simulink model "Scenario_2_v2"  (R2020b)
settings: Solver=ode1  StartTime=0.0  StopTime=10  FixedStep=Ts  MaxStep=Ts*2  MinStep=Ts/5  RelTol=1e-3
values from neighbouring files (symbols this model uses):
  c0 = c0_zeb    (= 6.57988e-09)    [Scenario_17_parameters_v2.m]    (also in Scenario_1_parameters_v2.m; Scenario_2_parameters_v2.m; Scenario_3_parameters_v2.m)
  c1 = c1_zeb    (= 9.15905e-09)    [Scenario_17_parameters_v2.m]    (also in Scenario_1_parameters_v2.m; Scenario_2_parameters_v2.m; Scenario_3_parameters_v2.m)
  fg = 50    [Scenario_17_parameters_v2.m]    (also in Scenario_1_parameters_v2.m; Scenario_2_parameters_v2.m; Scenario_3_parameters_v2.m)
  G1gen = 0.4692    [Scenario_17_parameters_v2.m]    (also in Scenario_1_parameters_v2.m = 0.1; Scenario_2_parameters_v2.m = 0.298581; Scenario_3_parameters_v2.m = 0.65)
  G2gen = 0.80    (= 0.8)    [Scenario_1_parameters_v2.m]    (also in Scenario_2_parameters_v2.m = 0.7; Scenario_3_parameters_v2.m = 0.4)
  G3gen = 0.85    [Scenario_1_parameters_v2.m]    (also in Scenario_2_parameters_v2.m = 0.9; Scenario_3_parameters_v2.m = 0.6)
  G4sgen = 0.8186    [Scenario_2_parameters_v2.m]
  G5gen = 0.75    [Scenario_17_parameters_v2.m]    (also in Scenario_1_parameters_v2.m = 0.8; Scenario_2_parameters_v2.m = 0.8; Scenario_3_parameters_v2.m = 0.705)
  G6gen = 0.90    (= 0.9)    [Scenario_17_parameters_v2.m]    (also in Scenario_1_parameters_v2.m; Scenario_2_parameters_v2.m = 0.81797; Scenario_3_parameters_v2.m = 0.45)
  G6sgen = 0.7    [Scenario_2_parameters_v2.m]
  G7gen = 0.20    (= 0.2)    [Scenario_17_parameters_v2.m]    (also in Scenario_1_parameters_v2.m = 0.5227; Scenario_2_parameters_v2.m = 0.5098; Scenario_3_parameters_v2.m = 0.4)
  Iovc = 1.2    [Scenario_17_parameters_v2.m]    (also in Scenario_1_parameters_v2.m; Scenario_2_parameters_v2.m; Scenario_3_parameters_v2.m)
  l0 = l0_zeb    (= 0.00368)    [Scenario_17_parameters_v2.m]    (also in Scenario_1_parameters_v2.m; Scenario_2_parameters_v2.m; Scenario_3_parameters_v2.m)
  l1 = l1_zeb    (= 0.00128)    [Scenario_17_parameters_v2.m]    (also in Scenario_1_parameters_v2.m; Scenario_2_parameters_v2.m; Scenario_3_parameters_v2.m)
  L3dem = 0.30    (= 0.3)    [Scenario_17_parameters_v2.m]    (also in Scenario_1_parameters_v2.m = 0.1; Scenario_2_parameters_v2.m = 0.1; Scenario_3_parameters_v2.m = 0.2)
  L4dem = 0.30    (= 0.3)    [Scenario_1_parameters_v2.m]    (also in Scenario_2_parameters_v2.m)
  L5dem = 0.25    [Scenario_17_parameters_v2.m]    (also in Scenario_1_parameters_v2.m = 0.35; Scenario_2_parameters_v2.m = 0.35; Scenario_3_parameters_v2.m = 0.1)
  L6dem = 0.15    [Scenario_1_parameters_v2.m]    (also in Scenario_2_parameters_v2.m; Scenario_3_parameters_v2.m = 0.1)
  L7dem = 0.10    (= 0.1)    [Scenario_1_parameters_v2.m]    (also in Scenario_2_parameters_v2.m; Scenario_3_parameters_v2.m = 0.2)
  Pr = Sr*PF    (= 1600500000)    [Scenario_17_parameters_v2.m]    (also in Scenario_1_parameters_v2.m = 1472500000; Scenario_2_parameters_v2.m = 1805000000; Scenario_3_parameters_v2.m = 12740000000)
  Qr = sqrt(Sr^2 - Pr^2)    [Scenario_17_parameters_v2.m]    (also in Scenario_1_parameters_v2.m; Scenario_2_parameters_v2.m; Scenario_3_parameters_v2.m)
  r0 = r0_zeb    (= 0.39362)    [Scenario_17_parameters_v2.m]    (also in Scenario_1_parameters_v2.m; Scenario_2_parameters_v2.m; Scenario_3_parameters_v2.m)
  r1 = r1_zeb    (= 0.06862)    [Scenario_17_parameters_v2.m]    (also in Scenario_1_parameters_v2.m; Scenario_2_parameters_v2.m; Scenario_3_parameters_v2.m)
  Rtpu = Xtpu/40    (= 0.0025)    [Scenario_17_parameters_v2.m]    (also in Scenario_1_parameters_v2.m = 0.00375; Scenario_2_parameters_v2.m = 0.00375; Scenario_3_parameters_v2.m)
  S1non = 700e6    (= 700000000)    [Scenario_17_parameters_v2.m]    (also in Scenario_1_parameters_v2.m = 400000000; Scenario_2_parameters_v2.m = 400000000; Scenario_3_parameters_v2.m = 1000000000)
  S2non = 300e6    (= 300000000)    [Scenario_1_parameters_v2.m]    (also in Scenario_2_parameters_v2.m; Scenario_3_parameters_v2.m = 3000000000)
  S3non = 200e6    (= 200000000)    [Scenario_1_parameters_v2.m]    (also in Scenario_2_parameters_v2.m; Scenario_3_parameters_v2.m = 1000000000)
  S4snon = 200e6    (= 200000000)    [Scenario_2_parameters_v2.m]
  S5non = 400e6    (= 400000000)    [Scenario_17_parameters_v2.m]    (also in Scenario_1_parameters_v2.m = 500000000; Scenario_2_parameters_v2.m = 500000000; Scenario_3_parameters_v2.m = 2000000000)
  S6non = 150e6    (= 150000000)    [Scenario_17_parameters_v2.m]    (also in Scenario_1_parameters_v2.m = 400000000; Scenario_2_parameters_v2.m = 400000000; Scenario_3_parameters_v2.m = 3000000000)
  S6snon = 200e6    (= 200000000)    [Scenario_2_parameters_v2.m]
  S7non = 1500e6    (= 1500000000)    [Scenario_17_parameters_v2.m]    (also in Scenario_1_parameters_v2.m = 200000000; Scenario_2_parameters_v2.m = 200000000; Scenario_3_parameters_v2.m = 4000000000)
  tonvsc = 0    [Scenario_17_parameters_v2.m]    (also in Scenario_1_parameters_v2.m; Scenario_2_parameters_v2.m; Scenario_3_parameters_v2.m = 0.0001)
  Ts = 50e-6    (= 5e-05)    [Scenario_17_parameters_v2.m]    (also in Scenario_1_parameters_v2.m = 0.0002; Scenario_2_parameters_v2.m = 2e-05; Scenario_3_parameters_v2.m = 0.0001)
  Vhv = 220e3    (= 220000)    [Scenario_17_parameters_v2.m]    (also in Scenario_1_parameters_v2.m; Scenario_2_parameters_v2.m; Scenario_3_parameters_v2.m)
  Vmv = 22e3    (= 22000)    [Scenario_17_parameters_v2.m]    (also in Scenario_1_parameters_v2.m; Scenario_2_parameters_v2.m; Scenario_3_parameters_v2.m)
  w_pll = 2*pi*80    (= 502.654824574)    [Scenario_17_parameters_v2.m]    (also in Scenario_1_parameters_v2.m; Scenario_2_parameters_v2.m; Scenario_3_parameters_v2.m)
  wc1 = wsw1/10    (= 848.230016469)    [Scenario_17_parameters_v2.m]    (also in Scenario_1_parameters_v2.m; Scenario_2_parameters_v2.m; Scenario_3_parameters_v2.m)
  wdc1 = wc1/10    (= 84.8230016469)    [Scenario_17_parameters_v2.m]    (also in Scenario_1_parameters_v2.m; Scenario_2_parameters_v2.m; Scenario_3_parameters_v2.m)
  wpq1 = wc1/10    (= 84.8230016469)    [Scenario_17_parameters_v2.m]    (also in Scenario_1_parameters_v2.m; Scenario_2_parameters_v2.m; Scenario_3_parameters_v2.m)
  wsw1 = ksw1*2*pi*fg    (= 8482.30016469)    [Scenario_17_parameters_v2.m]    (also in Scenario_1_parameters_v2.m; Scenario_2_parameters_v2.m; Scenario_3_parameters_v2.m)
  Xtpu = 0.10    (= 0.1)    [Scenario_17_parameters_v2.m]    (also in Scenario_1_parameters_v2.m = 0.15; Scenario_2_parameters_v2.m = 0.15; Scenario_3_parameters_v2.m)
undefined symbols (not defined in the file or in its folder): D11, Delta, Newton, Raphson
libraries: powerlib x214, simulink_extras x133, powerlib_meascontrol x102, pid_lib x48, simulink x32, eeTransforms x24, spsFirstOrderFilterLib x16, eePwmGeneratorTwoLevel x4
(part 2 of 19)

== system Scenario_2_v2/G2 ==
  Bus Selector : BusSelector  OutputSignals=Pabc,Qabc,vqp,vdp,vqn,vdn,iqp,idp,iqn,idn,f
  Constant : Constant  Value=S2non*G2gen
  Constant1 : Constant  Value=50e6
  Goto1 : Goto  Commented=on  GotoTag=Pg2  TagVisibility=global
  Goto3 : Goto  Commented=on  GotoTag=vdqpng2  TagVisibility=global
  Goto4 : Goto  Commented=on  GotoTag=idqpng2  TagVisibility=global
  Goto5 : Goto  Commented=on  GotoTag=Qg2  TagVisibility=global
  Mux2 : Mux
  Mux3 : Mux
  VSC v2 : Subsystem  mask{vscmod=EMT Average, fg=fg, Vhv=Vhv, Vmv=Vmv, Pconv=S2non, Rtpu=Rtpu, Xtpu=Xtpu, qmode=Active power, dmode=Reactive power, wsw=wsw1, wn_pll=w_pll, wc=wc1, wpq=wpq1, wdc=wdc1, koc=Iovc, Cdc=3100e-6, tfilt=1*(1/wsw1), negseq_en=on, fdroop_en=off, Vacdroop_en=off, LVRT_en=off, Kfdroop=0.05, fdroop_per=10, Kvdroop=0.1, Vacdroop_per=10, Vlvrt0=0.9, Vlvrt_min=0.5, Qmax_lvrt=0.9, V0pu=0.9540, theta0=-32.40, P0=S2non*G2gen, Q0=50e6}
      mask prompts: vscmod "VSC Model"; fg "AC grid frequency (Hz)"; Vhv "Grid-side voltage (V)(LL-rms)"; Vmv "Converter-side voltage (V)(LL-rms)"; Pconv "Converter nominal power (VA)"; Rtpu "Resistance seen by the converter (p.u)"; Xtpu "Reactance seen by the converter (p.u)"; qmode "q-axis control mode"; dmode "d-axis control mode"; wsw "Switching frequency (rad/s)"; wn_pll "PLL filter natural frequency"; wc "Current-control bandwidth (rad/s)"; wpq "PQ control bandwidth (rad/s)"; wdc "DC Voltage control bandwidth(rad/s)"; koc "Overcurrent factor (p.u)"; Cdc "DC-side total capacitance (F)"; tfilt "Vabc filter time constant (s)"; negseq_en "Enable negative sequence control"; fdroop_en "Enable frequency droop"; Vacdroop_en "Enable AC voltage droop"; LVRT_en "Enable LVRT"; Kfdroop "Frequency droop (p.u)"; fdroop_per "Percentage of converter power to contribute with droop (%)"; Kvdroop "Voltage droop (p.u)"; Vacdroop_per "Percentage of converter power to contribute with droop (%)"; Vlvrt0 "initial voltage (p.u)"; Vlvrt_min "minimum voltage (p.u)"; Qmax_lvrt "max power injected at min voltage (p.u)"; V0pu "Initial terminal voltage magnitude (pu)"; theta0 "Initial terminal voltage angle (deg)"; P0 "Initial active power (W)"; Q0 "Initial reactive power (VAr)"
      mask init:
      | %% ----------------------VSC Parameters-------------------------- %%
      | j = 1i;
      | r = Vhv/Vmv;                    % Transformer ratio
      | Vmvpk = Vmv*sqrt(2)/sqrt(3);    % Converter-side voltage phase-to-ground peak-to-peak
      | Vhvpk = Vhv*sqrt(2)/sqrt(3);    % Grid-side voltage phase-to-ground peak-to-peak  
      | Vdc = 2*Vhvpk;                  % Nominal DC voltage 
      | ksw = round(wsw/(2*pi*fg));      % Calculates switching ratio
      | Iconvbase = 2*Pconv/(3*Vmvpk);  % Converter base current (A)
      | Zbmv = Vmv^2/Pconv;             % Base voltage referred to the converter side
      | Imax = koc*Iconvbase;   % Converter maximum output current
      | %Cdc = 2*Hvsc*Pconv/Vdc^2;       % DC capacitor
      | 
      | Xt = Xtpu*Zbmv;        % p.u to (Ohms)
      | Lt = Xt/(2*pi*fg);              % p.u to (H)
      | Rt = Rtpu*Zbmv;        % p.u. to (Ohms)
      | 
      | % -------------LVRT--------------%
      | Klvrt = Qmax_lvrt/(Vlvrt_min-Vlvrt0); % Defines LVRT inclination of the V/I LVRT characteristic
      | 
      | % ------------ PLL ------------- %
      | zeta_pll = 1/sqrt(2);           % Damping
      | kp_pll = 2*zeta_pll*wn_pll/(Vmvpk);
      | tau_pll = 2*zeta_pll/wn_pll;
      | 
      | % ------------ Inner-loop (current control) ------------ %
      | kp_c = Lt*wc; 
      | ti_c = Lt/Rt;
      | 
      | % -------- Outer-loop (voltage and/or power control)
      | % --- PQ closed-loop control ----
      | ti_pq = 1/wc;
      | kp_pq = 2/3*ti_pq*wpq*1/Vmvpk;
      | 
      | % --- Vdc control ----
      | damp_dc = 1/sqrt(2);
      | kp_dc = 2*Cdc*damp_dc*wdc; 
      | ki_dc = Cdc*wdc^2;
      | 
      | %% ---------------------Mask operations----------------------------%%
      | 
      | % If the box is unchecked, we set the bias value to zero
      | if ~fdroop_en; end
      | if ~Vacdroop_en; end
      | if ~LVRT_en; Klvrt = 0;  end
      | 
      | %% -------------------- Variant Subsystem ----------------------- %%
      | choice = get_param(gcb,'vscmod'); % Get choice from list
      | VSS_model = [gcb, '/VSC Model'];  % VSC electrical Model
      | VSS_meas = [gcb, '/VSC Control/Measurements']; % Measurements (PLL, Park transformation, etc)
      | VSS_mod = [gcb, '/VSC Control/Modulation']; % Modulation or reference voltage/current generation
      | VSS_ctr = [gcb, '/VSC Control/Control loops']; % Modulation or reference voltage/current generation
      | 
      | 
      | if strcmp(choice,'EMT Switching')
      |     set_param(VSS_model, 'LabelModeActiveChoice', 'EMT_SW');
      |     set_param(VSS_meas, 'LabelModeActiveChoice', 'EMT');
      |     set_param(VSS_mod, 'LabelModeActiveChoice', 'EMT_SW');
      |     set_param(VSS_ctr, 'LabelModeActiveChoice', 'EMT_and_QEMT');
      |     
      | elseif strcmp(choice,'EMT Average')
      |     set_param(VSS_model, 'LabelModeActiveChoice', 'EMT_AVG');
      |     set_param(VSS_meas, 'LabelModeActiveChoice', 'EMT');
      |     set_param(VSS_mod, 'LabelModeActiveChoice', 'EMT_AVG');
      |     set_param(VSS_ctr, 'LabelModeActiveChoice', 'EMT_and_QEMT');
      |     %set_param([VSS_meas '/EMT/Vabc filter'],'Commented','through')
      |     tfilt = 0; % No filtering in Average model
      |     
      | elseif strcmp(choice,'Phasor Quasi-EMT')
      |     set_param(VSS_model, 'LabelModeActiveChoice', 'Phasor');
      |     set_param(VSS_meas, 'LabelModeActiveChoice', 'Phasor');
      |     set_param(VSS_mod, 'LabelModeActiveChoice', 'Phasor_QEMT');
      |     set_param(VSS_ctr, 'LabelModeActiveChoice', 'EMT_and_QEMT');
      |     
      | elseif strcmp(choice,'Phasor I-1st')
      |     set_param(VSS_model, 'LabelModeActiveChoice', 'Phasor');
      |     set_param(VSS_meas, 'LabelModeActiveChoice', 'Phasor');
      |     set_param(VSS_mod, 'LabelModeActiveChoice', 'Phasor_I_and_PQ');
      |     set_param(VSS_ctr, 'LabelModeActiveChoice', 'Phasor_I_1st');
      |     
      | elseif strcmp(choice,'Phasor I-ref')
      |     set_param(VSS_model, 'LabelModeActiveChoice', 'Phasor');
      | 	set_param(VSS_meas, 'LabelModeActiveChoice', 'Phasor');
      |     set_param(VSS_mod, 'LabelModeActiveChoice', 'Phasor_I_and_PQ');
      |     set_param(VSS_ctr, 'LabelModeActiveChoice', 'Phasor_I_ref');
      |     
      | elseif strcmp(choice,'Phasor PQ-1st')
      |     set_param(VSS_model, 'LabelModeActiveChoice', 'Phasor');
      |     set_param(VSS_meas, 'LabelModeActiveChoice', 'Phasor');
      |     set_param(VSS_mod, 'LabelModeActiveChoice', 'Phasor_I_and_PQ');
      |     set_param(VSS_ctr, 'LabelModeActiveChoice', 'Phasor_PQ');
      | end
      | 
      | 
      | %% ------------------------- Converter initialization -----------------------------
      | 
      | %-------------- Electrical part ----------------------
      | theta0 = theta0*pi/180; % deg to rad
      | 
      | Vgmag = V0pu*Vhv/sqrt(3); % Phase Voltage magnitude (LG,RMS)
      | Xt = Xtpu*Zbmv; % Converting the reactance the converter sees to Ohms
      | 
      | % Grid voltage in rectangular format, with reference to the MV-side (divided by the transformer relation)
      | [Vgr,Vgi] = pol2cart(theta0,Vgmag/r);
      | Vg = complex(Vgr,Vgi);
      | 
      | % Complex power
      | S0 = complex(P0,Q0);
      | 
      | % Converter output current (RMS), with reference to the MV side
      | Ic = conj(S0/(3*Vg));
      | 
      | % Converter internal voltage (LG,RMS), with reference to the MV side
      | Vc = Vg + Ic*(Rt + j*Xt);
      | 
      | %------------------- Converter part ----------------
      | 
      | % ---------- PLL -----------
      | % The angle used in dq transformation is different in EMT and in Phasor
      | if (strcmp(choice,'EMT Switching') || strcmp(choice,'EMT Average'))
      |     thetaPLL = pi + theta0;
      | elseif (strcmp(choice,'Phasor Quasi-EMT') || strcmp(choice,'Phasor I-1st') || strcmp(choice,'Phasor I-ref') || strcmp(choice,'Phasor PQ-1st'))
      |     thetaPLL = pi;
      | end
      | 
      | 
      | % ------ dq variables --------
      | 
      | Vgq = imag(Vg*sqrt(2)*exp(-j*(thetaPLL + pi/2))); 
      | Vgd = real(Vg*sqrt(2)*exp(-j*(thetaPLL + pi/2))); 
      | 
      | Vcq = imag(Vc*sqrt(2)*exp(-j*(thetaPLL + pi/2))); 
      | Vcd = real(Vc*sqrt(2)*exp(-j*(thetaPLL + pi/2))); 
      | 
      | Icq = imag(Ic*sqrt(2)*exp(-j*(thetaPLL + pi/2))); 
      | Icd = real(Ic*sqrt(2)*exp(-j*(thetaPLL + pi/2))); 
      | 
      | % ------ Inner loop ------
      | % Now that we know the reference voltage in dq (Vc,qd), the grid voltage in dq (Vg,qd) and the converter
      | % current in dq (Ic,dq), we can calculate the PI controller output in t=0
      | % As we assume zero steady-state error, the proportional part is zero and we calculate only the integrator part (Tc,qd)
      | Tcq = Vcq - Vgq - Xt*Icd;
      | Tcd = Vcd - Vgd + Xt*Icq;
      | 
      | % ------- Outer loop -------
      | % As we know the converter current, and we know that the proportional part is zero, we calculate the
      | % integrator part (To,qd)
      | Toq = Icq;
      | Tod = Icd;
      mask TypeOptions vscmod: EMT Switching | EMT Average | Phasor Quasi-EMT | Phasor I-1st | Phasor I-ref | Phasor PQ-1st
      mask Callback vscmod:
      | % Control parameter visiblity
      | 
      | % Get the value of the Enable Bias checkbox
      | % unchecked = 'off'
      | % checked = 'on'
      | 
      | maskObj = Simulink.Mask.get(gcb);
      | 
      | wn_pll = 'on';
      | wsw = 'on';
      | DC_en = 'off';
      | 
      | vscmod = get_param(gcb,'vscmod');
      |     if strcmp(vscmod,'EMT Switching')
      |       wn_pll = 'on';
      |       wsw = 'on';
      |       tfilt = 'on';
      |     elseif strcmp(vscmod,'EMT Average')
      |         wn_pll = 'on';
      |         wsw = 'off';
      |         tfilt = 'off';
      |     elseif strcmp(vscmod,'Phasor Quasi-EMT')
      |         wn_pll = 'off';
      |         wsw = 'off';
      |         tfilt = 'off';
      |     elseif strcmp(vscmod,'Phasor I-1st')
      |         wn_pll = 'off';
      |         wsw = 'off';
      |         tfilt = 'off';
      |     elseif strcmp(vscmod,'Phasor I-ref')
      |         wn_pll = 'off';
      |         wsw = 'off';
      |         tfilt = 'off';
      |     elseif strcmp(vscmod,'Phasor PQ-1st')
      |         wn_pll = 'off';
      |         wsw = 'off';
      |         tfilt = 'off';
      |     end
      | 
      | fdroop_en = get_param(gcb,'fdroop_en');
      | Vacdroop_en = get_param(gcb,'Vacdroop_en');
      | LVRT_en = get_param(gcb,'LVRT_en');
      | negseq_en = get_param(gcb,'negseq_en');
      | qmode_str = get_param(gcb,'qmode');
      | 
      | 
      | if strcmp(qmode_str,'DC voltage')
      |     DC_en = 'on';
      | else
      |     DC_en = 'off';
      | end
      | 
      | % Set the 'MaskVisibilities' property for each parameters
      |     set_param(gcb,'MaskVisibilities',{'on','on','on','on','on','on','on','on','on',wsw,wn_pll,'on','on','on','on',DC_en,tfilt,'on','on','on','on',fdroop_en,fdroop_en,Vacdroop_en,Vacdroop_en,'on','on','on','on','on','on','on'});
      | 
      | % Make LVRT area visible when it is enabled
      | if strcmp(LVRT_en,'on')
      |   maskObj.getDialogControl('Container_LVRT').Visible = 'on';
      | else
      |     maskObj.getDialogControl('Container_LVRT').Visible = 'off';
      | end
      | 
      | % Note that the value of the bias is not handled here.
      | % See the Initialization tab
      mask TypeOptions qmode: Active power | DC voltage
      mask Callback qmode:
      | % Control parameter visiblity
      | 
      | % Get the value of the Enable Bias checkbox
      | % unchecked = 'off'
      | % checked = 'on'
      | 
      | maskObj = Simulink.Mask.get(gcb);
      | 
      | wn_pll = 'on';
      | wsw = 'on';
      | DC_en = 'off';
      | 
      | vscmod = get_param(gcb,'vscmod');
      |     if strcmp(vscmod,'EMT Switching')
      |       wn_pll = 'on';
      |       wsw = 'on';
      |       tfilt = 'on';
      |     elseif strcmp(vscmod,'EMT Average')
      |         wn_pll = 'on';
      |         wsw = 'off';
      |         tfilt = 'off';
      |     elseif strcmp(vscmod,'Phasor Quasi-EMT')
      |         wn_pll = 'off';
      |         wsw = 'off';
      |         tfilt = 'off';
      |     elseif strcmp(vscmod,'Phasor I-1st')
      |         wn_pll = 'off';
      |         wsw = 'off';
      |         tfilt = 'off';
      |     elseif strcmp(vscmod,'Phasor I-ref')
      |         wn_pll = 'off';
      |         wsw = 'off';
      |         tfilt = 'off';
      |     elseif strcmp(vscmod,'Phasor PQ-1st')
      |         wn_pll = 'off';
      |         wsw = 'off';
      |         tfilt = 'off';
      |     end
      | 
      | fdroop_en = get_param(gcb,'fdroop_en');
      | Vacdroop_en = get_param(gcb,'Vacdroop_en');
      | LVRT_en = get_param(gcb,'LVRT_en');
      | negseq_en = get_param(gcb,'negseq_en');
      | qmode_str = get_param(gcb,'qmode');
      | 
      | 
      | if strcmp(qmode_str,'DC voltage')
      |     DC_en = 'on';
      | else
      |     DC_en = 'off';
      | end
      | 
      | % Set the 'MaskVisibilities' property for each parameters
      |     set_param(gcb,'MaskVisibilities',{'on','on','on','on','on','on','on','on','on',wsw,wn_pll,'on','on','on','on',DC_en,tfilt,'on','on','on','on',fdroop_en,fdroop_en,Vacdroop_en,Vacdroop_en,'on','on','on','on','on','on','on'});
      | 
      | % Make LVRT area visible when it is enabled
      | if strcmp(LVRT_en,'on')
      |   maskObj.getDialogControl('Container_LVRT').Visible = 'on';
      | else
      |     maskObj.getDialogControl('Container_LVRT').Visible = 'off';
      | end
      | 
      | % Note that the value of the bias is not handled here.
      | % See the Initialization tab
      mask TypeOptions dmode: Reactive power | AC voltage
      mask Callback fdroop_en:
      | % Control parameter visiblity
      | 
      | % Get the value of the Enable Bias checkbox
      | % unchecked = 'off'
      | % checked = 'on'
      | 
      | maskObj = Simulink.Mask.get(gcb);
      | 
      | wn_pll = 'on';
      | wsw = 'on';
      | DC_en = 'off';
      | 
      | vscmod = get_param(gcb,'vscmod');
      |     if strcmp(vscmod,'EMT Switching')
      |       wn_pll = 'on';
      |       wsw = 'on';
      |       tfilt = 'on';
      |     elseif strcmp(vscmod,'EMT Average')
      |         wn_pll = 'on';
      |         wsw = 'off';
      |         tfilt = 'off';
      |     elseif strcmp(vscmod,'Phasor Quasi-EMT')
      |         wn_pll = 'off';
      |         wsw = 'off';
      |         tfilt = 'off';
      |     elseif strcmp(vscmod,'Phasor I-1st')
      |         wn_pll = 'off';
      |         wsw = 'off';
      |         tfilt = 'off';
      |     elseif strcmp(vscmod,'Phasor I-ref')
      |         wn_pll = 'off';
      |         wsw = 'off';
      |         tfilt = 'off';
      |     elseif strcmp(vscmod,'Phasor PQ-1st')
      |         wn_pll = 'off';
      |         wsw = 'off';
      |         tfilt = 'off';
      |     end
      | 
      | fdroop_en = get_param(gcb,'fdroop_en');
      | Vacdroop_en = get_param(gcb,'Vacdroop_en');
      | LVRT_en = get_param(gcb,'LVRT_en');
      | negseq_en = get_param(gcb,'negseq_en');
      | qmode_str = get_param(gcb,'qmode');
      | 
      | 
      | if strcmp(qmode_str,'DC voltage')
      |     DC_en = 'on';
      | else
      |     DC_en = 'off';
      | end
      | 
      | % Set the 'MaskVisibilities' property for each parameters
      |     set_param(gcb,'MaskVisibilities',{'on','on','on','on','on','on','on','on','on',wsw,wn_pll,'on','on','on','on',DC_en,tfilt,'on','on','on','on',fdroop_en,fdroop_en,Vacdroop_en,Vacdroop_en,'on','on','on','on','on','on','on'});
      | 
      | % Make LVRT area visible when it is enabled
      | if strcmp(LVRT_en,'on')
      |   maskObj.getDialogControl('Container_LVRT').Visible = 'on';
      | else
      |     maskObj.getDialogControl('Container_LVRT').Visible = 'off';
      | end
      | 
      | % Note that the value of the bias is not handled here.
      | % See the Initialization tab
      mask Callback Vacdroop_en:
      | % Control parameter visiblity
      | 
      | % Get the value of the Enable Bias checkbox
      | % unchecked = 'off'
      | % checked = 'on'
      | 
      | maskObj = Simulink.Mask.get(gcb);
      | 
      | wn_pll = 'on';
      | wsw = 'on';
      | DC_en = 'off';
      | 
      | vscmod = get_param(gcb,'vscmod');
      |     if strcmp(vscmod,'EMT Switching')
      |       wn_pll = 'on';
      |       wsw = 'on';
      |       tfilt = 'on';
      |     elseif strcmp(vscmod,'EMT Average')
      |         wn_pll = 'on';
      |         wsw = 'off';
      |         tfilt = 'off';
      |     elseif strcmp(vscmod,'Phasor Quasi-EMT')
      |         wn_pll = 'off';
      |         wsw = 'off';
      |         tfilt = 'off';
      |     elseif strcmp(vscmod,'Phasor I-1st')
      |         wn_pll = 'off';
      |         wsw = 'off';
      |         tfilt = 'off';
      |     elseif strcmp(vscmod,'Phasor I-ref')
      |         wn_pll = 'off';
      |         wsw = 'off';
      |         tfilt = 'off';
      |     elseif strcmp(vscmod,'Phasor PQ-1st')
      |         wn_pll = 'off';
      |         wsw = 'off';
      |         tfilt = 'off';
      |     end
      | 
      | fdroop_en = get_param(gcb,'fdroop_en');
      | Vacdroop_en = get_param(gcb,'Vacdroop_en');
      | LVRT_en = get_param(gcb,'LVRT_en');
      | negseq_en = get_param(gcb,'negseq_en');
      | qmode_str = get_param(gcb,'qmode');
      | 
      | 
      | if strcmp(qmode_str,'DC voltage')
      |     DC_en = 'on';
      | else
      |     DC_en = 'off';
      | end
      | 
      | % Set the 'MaskVisibilities' property for each parameters
      |     set_param(gcb,'MaskVisibilities',{'on','on','on','on','on','on','on','on','on',wsw,wn_pll,'on','on','on','on',DC_en,tfilt,'on','on','on','on',fdroop_en,fdroop_en,Vacdroop_en,Vacdroop_en,'on','on','on','on','on','on','on'});
      | 
      | % Make LVRT area visible when it is enabled
      | if strcmp(LVRT_en,'on')
      |   maskObj.getDialogControl('Container_LVRT').Visible = 'on';
      | else
      |     maskObj.getDialogControl('Container_LVRT').Visible = 'off';
      | end
      | 
      | % Note that the value of the bias is not handled here.
      | % See the Initialization tab
      mask Callback LVRT_en:
      | % Control parameter visiblity
      | 
      | % Get the value of the Enable Bias checkbox
      | % unchecked = 'off'
      | % checked = 'on'
      | 
      | maskObj = Simulink.Mask.get(gcb);
      | 
      | wn_pll = 'on';
      | wsw = 'on';
      | DC_en = 'off';
      | 
      | vscmod = get_param(gcb,'vscmod');
      |     if strcmp(vscmod,'EMT Switching')
      |       wn_pll = 'on';
      |       wsw = 'on';
      |       tfilt = 'on';
      |     elseif strcmp(vscmod,'EMT Average')
      |         wn_pll = 'on';
      |         wsw = 'off';
      |         tfilt = 'off';
      |     elseif strcmp(vscmod,'Phasor Quasi-EMT')
      |         wn_pll = 'off';
      |         wsw = 'off';
      |         tfilt = 'off';
      |     elseif strcmp(vscmod,'Phasor I-1st')
      |         wn_pll = 'off';
      |         wsw = 'off';
      |         tfilt = 'off';
      |     elseif strcmp(vscmod,'Phasor I-ref')
      |         wn_pll = 'off';
      |         wsw = 'off';
      |         tfilt = 'off';
      |     elseif strcmp(vscmod,'Phasor PQ-1st')
      |         wn_pll = 'off';
      |         wsw = 'off';
      |         tfilt = 'off';
      |     end
      | 
      | fdroop_en = get_param(gcb,'fdroop_en');
      | Vacdroop_en = get_param(gcb,'Vacdroop_en');
      | LVRT_en = get_param(gcb,'LVRT_en');
      | negseq_en = get_param(gcb,'negseq_en');
      | qmode_str = get_param(gcb,'qmode');
      | 
      | 
      | if strcmp(qmode_str,'DC voltage')
      |     DC_en = 'on';
      | else
      |     DC_en = 'off';
      | end
      | 
      | % Set the 'MaskVisibilities' property for each parameters
      |     set_param(gcb,'MaskVisibilities',{'on','on','on','on','on','on','on','on','on',wsw,wn_pll,'on','on','on','on',DC_en,tfilt,'on','on','on','on',fdroop_en,fdroop_en,Vacdroop_en,Vacdroop_en,'on','on','on','on','on','on','on'});
      | 
      | % Make LVRT area visible when it is enabled
      | if strcmp(LVRT_en,'on')
      |   maskObj.getDialogControl('Container_LVRT').Visible = 'on';
      | else
      |     maskObj.getDialogControl('Container_LVRT').Visible = 'off';
      | end
      | 
      | % Note that the value of the bias is not handled here.
      | % See the Initialization tab
      mask DialogControl DescTextVar Prompt: -------------------------------------Three-phase VSC model---------------------------------------
      mask DialogControl Tab1 Prompt: Electrical parameters
      mask DialogControl Tab2 Prompt: Control parameters
      mask DialogControl Tab3 Prompt: Other parameters
      mask DialogControl Container_LVRT Prompt: LVRT
      mask DialogControl Tab4 Prompt: Power flow
      mask Display:
      | choice = get_param(gcb,'vscmod');
      | if strcmp(choice,'Phasor Quasi-EMT')
      |     disp('VSC\n\n')
      |     disp('\n\nPhasor\n\n')
      |     disp('\n\nQuasi-EMT')
      | elseif strcmp(choice,'EMT Average')
      |     disp('VSC\n')
      |     disp('\nEMT AVG')
      | elseif strcmp(choice,'EMT Switching')
      |     disp('VSC\n')
      |     disp('\nEMT SW')
      | elseif strcmp(choice,'Phasor I-1st')
      |     disp('VSC\n\n')
      |     disp('\n\nPhasor\n\n')
      |     disp('\n\nI 1st')
      | elseif strcmp(choice,'Phasor I-ref')
      |     disp('VSC\n\n')
      |     disp('\n\nPhasor\n\n')
      |     disp('\n\nI ref')
      | elseif strcmp(choice,'Phasor PQ-1st')
      |     disp('VSC\n\n')
      |     disp('\n\nPhasor\n\n')
      |     disp('\n\nPQ 1st')
      | end
  A : PMIOPort  Side=Right
  B : PMIOPort  Port=2  Side=Right
  C : PMIOPort  Port=3  Side=Right
  tag scope: fg2=global
  wires:
  Bus Selector/9 -> Mux3/3  "<iqn>"
  Bus Selector/3 -> Mux2/1  "<vqp>"
  Bus Selector/4 -> Mux2/2  "<vdp>"
  Bus Selector/8 -> Mux3/2  "<idp>"
  Mux3/1 -> Goto4/1
  Bus Selector/10 -> Mux3/4  "<idn>"
  Mux2/1 -> Goto3/1
  Bus Selector/6 -> Mux2/4  "<vdn>"
  Bus Selector/7 -> Mux3/1  "<iqp>"
  VSC v2/1(m) -> Bus Selector/1
  Bus Selector/5 -> Mux2/3  "<vqn>"
  Bus Selector/11 -> [fg2]  "<f>"
  Bus Selector/1 -> Goto1/1  "<Pabc>"
  Bus Selector/2 -> Goto5/1  "<Qabc>"
  Constant/1 -> VSC v2/1(Pset)
  Constant1/1 -> VSC v2/2(Qset)
  connections:
  VSC v2/LConn2 -- B/RConn1
  VSC v2/LConn1 -- A/RConn1
  VSC v2/LConn3 -- C/RConn1

== system Scenario_2_v2/G3 ==
  Bus Selector : BusSelector  OutputSignals=Pabc,Qabc,vqp,vdp,vqn,vdn,iqp,idp,iqn,idn,f
  Constant : Constant  Value=S3non*G3gen
  Constant1 : Constant  Value=50e6
  Goto1 : Goto  Commented=on  GotoTag=Pg3  TagVisibility=global
  Goto3 : Goto  Commented=on  GotoTag=vdqpng3  TagVisibility=global
  Goto4 : Goto  Commented=on  GotoTag=idqpng3  TagVisibility=global
  Goto5 : Goto  Commented=on  GotoTag=Qg3  TagVisibility=global
  Mux2 : Mux
  Mux3 : Mux
  VSC v2 : Subsystem  mask{vscmod=EMT Average, fg=fg, Vhv=Vhv, Vmv=Vmv, Pconv=S3non, Rtpu=Rtpu, Xtpu=Xtpu, qmode=Active power, dmode=Reactive power, wsw=wsw1, wn_pll=w_pll, wc=wc1, wpq=wpq1, wdc=wdc1, koc=Iovc, Cdc=3100e-6, tfilt=1*(1/wsw1), negseq_en=off, fdroop_en=off, Vacdroop_en=off, LVRT_en=off, Kfdroop=0.05, fdroop_per=10, Kvdroop=0.1, Vacdroop_per=10, Vlvrt0=0.9, Vlvrt_min=0.5, Qmax_lvrt=0.9, V0pu=0.9480, theta0=-33.35, P0=S3non*G3gen, Q0=50e6}
      mask prompts: vscmod "VSC Model"; fg "AC grid frequency (Hz)"; Vhv "Grid-side voltage (V)(LL-rms)"; Vmv "Converter-side voltage (V)(LL-rms)"; Pconv "Converter nominal power (VA)"; Rtpu "Resistance seen by the converter (p.u)"; Xtpu "Reactance seen by the converter (p.u)"; qmode "q-axis control mode"; dmode "d-axis control mode"; wsw "Switching frequency (rad/s)"; wn_pll "PLL filter natural frequency"; wc "Current-control bandwidth (rad/s)"; wpq "PQ control bandwidth (rad/s)"; wdc "DC Voltage control bandwidth(rad/s)"; koc "Overcurrent factor (p.u)"; Cdc "DC-side total capacitance (F)"; tfilt "Vabc filter time constant (s)"; negseq_en "Enable negative sequence control"; fdroop_en "Enable frequency droop"; Vacdroop_en "Enable AC voltage droop"; LVRT_en "Enable LVRT"; Kfdroop "Frequency droop (p.u)"; fdroop_per "Percentage of converter power to contribute with droop (%)"; Kvdroop "Voltage droop (p.u)"; Vacdroop_per "Percentage of converter power to contribute with droop (%)"; Vlvrt0 "initial voltage (p.u)"; Vlvrt_min "minimum voltage (p.u)"; Qmax_lvrt "max power injected at min voltage (p.u)"; V0pu "Initial terminal voltage magnitude (pu)"; theta0 "Initial terminal voltage angle (deg)"; P0 "Initial active power (W)"; Q0 "Initial reactive power (VAr)"
      mask init: same as Scenario_2_v2/G2/VSC v2
      mask TypeOptions vscmod: EMT Switching | EMT Average | Phasor Quasi-EMT | Phasor I-1st | Phasor I-ref | Phasor PQ-1st
      mask Callback vscmod:
      | % Control parameter visiblity
      | 
      | % Get the value of the Enable Bias checkbox
      | % unchecked = 'off'
      | % checked = 'on'
      | 
      | maskObj = Simulink.Mask.get(gcb);
      | 
      | wn_pll = 'on';
      | wsw = 'on';
      | DC_en = 'off';
      | 
      | vscmod = get_param(gcb,'vscmod');
      |     if strcmp(vscmod,'EMT Switching')
      |       wn_pll = 'on';
      |       wsw = 'on';
      |       tfilt = 'on';
      |     elseif strcmp(vscmod,'EMT Average')
      |         wn_pll = 'on';
      |         wsw = 'off';
      |         tfilt = 'off';
      |     elseif strcmp(vscmod,'Phasor Quasi-EMT')
      |         wn_pll = 'off';
      |         wsw = 'off';
      |         tfilt = 'off';
      |     elseif strcmp(vscmod,'Phasor I-1st')
      |         wn_pll = 'off';
      |         wsw = 'off';
      |         tfilt = 'off';
      |     elseif strcmp(vscmod,'Phasor I-ref')
      |         wn_pll = 'off';
      |         wsw = 'off';
      |         tfilt = 'off';
      |     elseif strcmp(vscmod,'Phasor PQ-1st')
      |         wn_pll = 'off';
      |         wsw = 'off';
      |         tfilt = 'off';
      |     end
      | 
      | fdroop_en = get_param(gcb,'fdroop_en');
      | Vacdroop_en = get_param(gcb,'Vacdroop_en');
      | LVRT_en = get_param(gcb,'LVRT_en');
      | negseq_en = get_param(gcb,'negseq_en');
      | qmode_str = get_param(gcb,'qmode');
      | 
      | 
      | if strcmp(qmode_str,'DC voltage')
      |     DC_en = 'on';
      | else
      |     DC_en = 'off';
      | end
      | 
      | % Set the 'MaskVisibilities' property for each parameters
      |     set_param(gcb,'MaskVisibilities',{'on','on','on','on','on','on','on','on','on',wsw,wn_pll,'on','on','on','on',DC_en,tfilt,'on','on','on','on',fdroop_en,fdroop_en,Vacdroop_en,Vacdroop_en,'on','on','on','on','on','on','on'});
      | 
      | % Make LVRT area visible when it is enabled
      | if strcmp(LVRT_en,'on')
      |   maskObj.getDialogControl('Container_LVRT').Visible = 'on';
      | else
      |     maskObj.getDialogControl('Container_LVRT').Visible = 'off';
      | end
      | 
      | % Note that the value of the bias is not handled here.
      | % See the Initialization tab
      mask TypeOptions qmode: Active power | DC voltage
      mask Callback qmode:
      | % Control parameter visiblity
      | 
      | % Get the value of the Enable Bias checkbox
      | % unchecked = 'off'
      | % checked = 'on'
      | 
      | maskObj = Simulink.Mask.get(gcb);
      | 
      | wn_pll = 'on';
      | wsw = 'on';
      | DC_en = 'off';
      | 
      | vscmod = get_param(gcb,'vscmod');
      |     if strcmp(vscmod,'EMT Switching')
      |       wn_pll = 'on';
      |       wsw = 'on';
      |       tfilt = 'on';
      |     elseif strcmp(vscmod,'EMT Average')
      |         wn_pll = 'on';
      |         wsw = 'off';
      |         tfilt = 'off';
      |     elseif strcmp(vscmod,'Phasor Quasi-EMT')
      |         wn_pll = 'off';
      |         wsw = 'off';
      |         tfilt = 'off';
      |     elseif strcmp(vscmod,'Phasor I-1st')
      |         wn_pll = 'off';
      |         wsw = 'off';
      |         tfilt = 'off';
      |     elseif strcmp(vscmod,'Phasor I-ref')
      |         wn_pll = 'off';
      |         wsw = 'off';
      |         tfilt = 'off';
      |     elseif strcmp(vscmod,'Phasor PQ-1st')
      |         wn_pll = 'off';
      |         wsw = 'off';
      |         tfilt = 'off';
      |     end
      | 
      | fdroop_en = get_param(gcb,'fdroop_en');
      | Vacdroop_en = get_param(gcb,'Vacdroop_en');
      | LVRT_en = get_param(gcb,'LVRT_en');
      | negseq_en = get_param(gcb,'negseq_en');
      | qmode_str = get_param(gcb,'qmode');
      | 
      | 
      | if strcmp(qmode_str,'DC voltage')
      |     DC_en = 'on';
      | else
      |     DC_en = 'off';
      | end
      | 
      | % Set the 'MaskVisibilities' property for each parameters
      |     set_param(gcb,'MaskVisibilities',{'on','on','on','on','on','on','on','on','on',wsw,wn_pll,'on','on','on','on',DC_en,tfilt,'on','on','on','on',fdroop_en,fdroop_en,Vacdroop_en,Vacdroop_en,'on','on','on','on','on','on','on'});
      | 
      | % Make LVRT area visible when it is enabled
      | if strcmp(LVRT_en,'on')
      |   maskObj.getDialogControl('Container_LVRT').Visible = 'on';
      | else
      |     maskObj.getDialogControl('Container_LVRT').Visible = 'off';
      | end
      | 
      | % Note that the value of the bias is not handled here.
      | % See the Initialization tab
      mask TypeOptions dmode: Reactive power | AC voltage
      mask Callback fdroop_en:
      | % Control parameter visiblity
      | 
      | % Get the value of the Enable Bias checkbox
      | % unchecked = 'off'
      | % checked = 'on'
      | 
      | maskObj = Simulink.Mask.get(gcb);
      | 
      | wn_pll = 'on';
      | wsw = 'on';
      | DC_en = 'off';
      | 
      | vscmod = get_param(gcb,'vscmod');
      |     if strcmp(vscmod,'EMT Switching')
      |       wn_pll = 'on';
      |       wsw = 'on';
      |       tfilt = 'on';
      |     elseif strcmp(vscmod,'EMT Average')
      |         wn_pll = 'on';
      |         wsw = 'off';
      |         tfilt = 'off';
      |     elseif strcmp(vscmod,'Phasor Quasi-EMT')
      |         wn_pll = 'off';
      |         wsw = 'off';
      |         tfilt = 'off';
      |     elseif strcmp(vscmod,'Phasor I-1st')
      |         wn_pll = 'off';
      |         wsw = 'off';
      |         tfilt = 'off';
      |     elseif strcmp(vscmod,'Phasor I-ref')
      |         wn_pll = 'off';
      |         wsw = 'off';
      |         tfilt = 'off';
      |     elseif strcmp(vscmod,'Phasor PQ-1st')
      |         wn_pll = 'off';
      |         wsw = 'off';
      |         tfilt = 'off';
      |     end
      | 
      | fdroop_en = get_param(gcb,'fdroop_en');
      | Vacdroop_en = get_param(gcb,'Vacdroop_en');
      | LVRT_en = get_param(gcb,'LVRT_en');
      | negseq_en = get_param(gcb,'negseq_en');
      | qmode_str = get_param(gcb,'qmode');
      | 
      | 
      | if strcmp(qmode_str,'DC voltage')
      |     DC_en = 'on';
      | else
      |     DC_en = 'off';
      | end
      | 
      | % Set the 'MaskVisibilities' property for each parameters
      |     set_param(gcb,'MaskVisibilities',{'on','on','on','on','on','on','on','on','on',wsw,wn_pll,'on','on','on','on',DC_en,tfilt,'on','on','on','on',fdroop_en,fdroop_en,Vacdroop_en,Vacdroop_en,'on','on','on','on','on','on','on'});
      | 
      | % Make LVRT area visible when it is enabled
      | if strcmp(LVRT_en,'on')
      |   maskObj.getDialogControl('Container_LVRT').Visible = 'on';
      | else
      |     maskObj.getDialogControl('Container_LVRT').Visible = 'off';
      | end
      | 
      | % Note that the value of the bias is not handled here.
      | % See the Initialization tab
      mask Callback Vacdroop_en:
      | % Control parameter visiblity
      | 
      | % Get the value of the Enable Bias checkbox
      | % unchecked = 'off'
      | % checked = 'on'
      | 
      | maskObj = Simulink.Mask.get(gcb);
      | 
      | wn_pll = 'on';
      | wsw = 'on';
      | DC_en = 'off';
      | 
      | vscmod = get_param(gcb,'vscmod');
      |     if strcmp(vscmod,'EMT Switching')
      |       wn_pll = 'on';
      |       wsw = 'on';
      |       tfilt = 'on';
      |     elseif strcmp(vscmod,'EMT Average')
      |         wn_pll = 'on';
      |         wsw = 'off';
      |         tfilt = 'off';
      |     elseif strcmp(vscmod,'Phasor Quasi-EMT')
      |         wn_pll = 'off';
      |         wsw = 'off';
      |         tfilt = 'off';
      |     elseif strcmp(vscmod,'Phasor I-1st')
      |         wn_pll = 'off';
      |         wsw = 'off';
      |         tfilt = 'off';
      |     elseif strcmp(vscmod,'Phasor I-ref')
      |         wn_pll = 'off';
      |         wsw = 'off';
      |         tfilt = 'off';
      |     elseif strcmp(vscmod,'Phasor PQ-1st')
      |         wn_pll = 'off';
      |         wsw = 'off';
      |         tfilt = 'off';
      |     end
      | 
      | fdroop_en = get_param(gcb,'fdroop_en');
      | Vacdroop_en = get_param(gcb,'Vacdroop_en');
      | LVRT_en = get_param(gcb,'LVRT_en');
      | negseq_en = get_param(gcb,'negseq_en');
      | qmode_str = get_param(gcb,'qmode');
      | 
      | 
      | if strcmp(qmode_str,'DC voltage')
      |     DC_en = 'on';
      | else
      |     DC_en = 'off';
      | end
      | 
      | % Set the 'MaskVisibilities' property for each parameters
      |     set_param(gcb,'MaskVisibilities',{'on','on','on','on','on','on','on','on','on',wsw,wn_pll,'on','on','on','on',DC_en,tfilt,'on','on','on','on',fdroop_en,fdroop_en,Vacdroop_en,Vacdroop_en,'on','on','on','on','on','on','on'});
      | 
      | % Make LVRT area visible when it is enabled
      | if strcmp(LVRT_en,'on')
      |   maskObj.getDialogControl('Container_LVRT').Visible = 'on';
      | else
      |     maskObj.getDialogControl('Container_LVRT').Visible = 'off';
      | end
      | 
      | % Note that the value of the bias is not handled here.
      | % See the Initialization tab
      mask Callback LVRT_en:
      | % Control parameter visiblity
      | 
      | % Get the value of the Enable Bias checkbox
      | % unchecked = 'off'
      | % checked = 'on'
      | 
      | maskObj = Simulink.Mask.get(gcb);
      | 
      | wn_pll = 'on';
      | wsw = 'on';
      | DC_en = 'off';
      | 
      | vscmod = get_param(gcb,'vscmod');
      |     if strcmp(vscmod,'EMT Switching')
      |       wn_pll = 'on';
      |       wsw = 'on';
      |       tfilt = 'on';
      |     elseif strcmp(vscmod,'EMT Average')
      |         wn_pll = 'on';
      |         wsw = 'off';
      |         tfilt = 'off';
      |     elseif strcmp(vscmod,'Phasor Quasi-EMT')
      |         wn_pll = 'off';
      |         wsw = 'off';
      |         tfilt = 'off';
      |     elseif strcmp(vscmod,'Phasor I-1st')
      |         wn_pll = 'off';
      |         wsw = 'off';
      |         tfilt = 'off';
      |     elseif strcmp(vscmod,'Phasor I-ref')
      |         wn_pll = 'off';
      |         wsw = 'off';
      |         tfilt = 'off';
      |     elseif strcmp(vscmod,'Phasor PQ-1st')
      |         wn_pll = 'off';
      |         wsw = 'off';
      |         tfilt = 'off';
      |     end
      | 
      | fdroop_en = get_param(gcb,'fdroop_en');
      | Vacdroop_en = get_param(gcb,'Vacdroop_en');
      | LVRT_en = get_param(gcb,'LVRT_en');
      | negseq_en = get_param(gcb,'negseq_en');
      | qmode_str = get_param(gcb,'qmode');
      | 
      | 
      | if strcmp(qmode_str,'DC voltage')
      |     DC_en = 'on';
      | else
      |     DC_en = 'off';
      | end
      | 
      | % Set the 'MaskVisibilities' property for each parameters
      |     set_param(gcb,'MaskVisibilities',{'on','on','on','on','on','on','on','on','on',wsw,wn_pll,'on','on','on','on',DC_en,tfilt,'on','on','on','on',fdroop_en,fdroop_en,Vacdroop_en,Vacdroop_en,'on','on','on','on','on','on','on'});
      | 
      | % Make LVRT area visible when it is enabled
      | if strcmp(LVRT_en,'on')
      |   maskObj.getDialogControl('Container_LVRT').Visible = 'on';
      | else
      |     maskObj.getDialogControl('Container_LVRT').Visible = 'off';
      | end
      | 
      | % Note that the value of the bias is not handled here.
      | % See the Initialization tab
      mask DialogControl DescTextVar Prompt: -------------------------------------Three-phase VSC model---------------------------------------
      mask DialogControl Tab1 Prompt: Electrical parameters
      mask DialogControl Tab2 Prompt: Control parameters
      mask DialogControl Tab3 Prompt: Other parameters
      mask DialogControl Container_LVRT Prompt: LVRT
      mask DialogControl Tab4 Prompt: Power flow
      mask Display:
      | choice = get_param(gcb,'vscmod');
      | if strcmp(choice,'Phasor Quasi-EMT')
      |     disp('VSC\n\n')
      |     disp('\n\nPhasor\n\n')
      |     disp('\n\nQuasi-EMT')
      | elseif strcmp(choice,'EMT Average')
      |     disp('VSC\n')
      |     disp('\nEMT AVG')
      | elseif strcmp(choice,'EMT Switching')
      |     disp('VSC\n')
      |     disp('\nEMT SW')
      | elseif strcmp(choice,'Phasor I-1st')
      |     disp('VSC\n\n')
      |     disp('\n\nPhasor\n\n')
      |     disp('\n\nI 1st')
      | elseif strcmp(choice,'Phasor I-ref')
      |     disp('VSC\n\n')
      |     disp('\n\nPhasor\n\n')
      |     disp('\n\nI ref')
      | elseif strcmp(choice,'Phasor PQ-1st')
      |     disp('VSC\n\n')
      |     disp('\n\nPhasor\n\n')
      |     disp('\n\nPQ 1st')
      | end
  A : PMIOPort  Side=Right
  B : PMIOPort  Port=2  Side=Right
  C : PMIOPort  Port=3  Side=Right
  tag scope: fg3=global
  wires:
  Bus Selector/11 -> [fg3]  "<f>"
  Bus Selector/5 -> Mux2/3  "<vqn>"
  VSC v2/1(m) -> Bus Selector/1
  Bus Selector/7 -> Mux3/1  "<iqp>"
  Bus Selector/6 -> Mux2/4  "<vdn>"
  Mux2/1 -> Goto3/1
  Bus Selector/10 -> Mux3/4  "<idn>"
  Mux3/1 -> Goto4/1
  Bus Selector/8 -> Mux3/2  "<idp>"
  Bus Selector/1 -> Goto1/1  "<Pabc>"
  Bus Selector/4 -> Mux2/2  "<vdp>"
  Bus Selector/3 -> Mux2/1  "<vqp>"
  Bus Selector/9 -> Mux3/3  "<iqn>"
  Bus Selector/2 -> Goto5/1  "<Qabc>"
  Constant/1 -> VSC v2/1(Pset)
  Constant1/1 -> VSC v2/2(Qset)
  connections:
  VSC v2/LConn3 -- C/RConn1
  A/RConn1 -- VSC v2/LConn1
  VSC v2/LConn2 -- B/RConn1
